simulink model "ADMIRE"  (R2021b)
settings: Solver=ode4  StartTime=0.0  StopTime=100  FixedStep=1e-2  RelTol=1e-3
undefined symbols (not defined in the file or in its folder): admireDB, Earth, WGS84
libraries: simulink_extras x112, simulink x27, aerolibutil x4, dspsigops x4, aerolibfltsims x3, sharedtransform x2, aerolibtransform2 x2, aerolibatmos2 x1, matrix_library x1, sharedutil x1, aerolibanimutils x1, vrlib x1
(part 13 of 15)

== system ADMIRE/Aircraft/Aerodynamics/RollMomentCoefficient/MachRegion3/Crmdr/Crmdr_ ==
  qacorr : Inport
  mach_nd : Inport  Port=2
  dR : Inport  Port=3
  CRMDRM_M : Lookup_n-D  NumberOfTableDimensions=1  BreakpointsForDimension1=admireDB.aerodata_asym_ext.CRMDRM.breakpoints.M  BreakpointsForDimension3=[5, 7]  Table=admireDB.aerodata_asym_ext.CRMDRM.newTable  ExtrapMethod=Clip  InternalRulePriority=Speed  RndMeth=Simplest  InputSameDT=on
  CRMEDR_QA_M : Lookup_n-D  BreakpointsForDimension1=admireDB.aerodata_asym_ext.CRMEDR.breakpoints.M  BreakpointsForDimension2=admireDB.aerodata_asym_ext.CRMEDR.breakpoints.QA  BreakpointsForDimension3=[5, 7]  Table=admireDB.aerodata_asym_ext.CRMEDR.newTable  ExtrapMethod=Clip  InternalRulePriority=Speed  RndMeth=Simplest  InputSameDT=on
      settings: InputPortMap=u0,u1
  Degrees to Radians : simulink_extras/Transformations/Degrees to Radians
  Product2 : Product  Inputs=3
  Crmdr : Outport
  wires:
  dR/1 -> Degrees to Radians/1
  CRMDRM_M/1 -> Product2/1
  Degrees to Radians/1 -> Product2/2
  qacorr/1 -> CRMEDR_QA_M/2
  mach_nd/1 -> CRMEDR_QA_M/1, CRMDRM_M/1
  CRMEDR_QA_M/1 -> Product2/3
  Product2/1 -> Crmdr/1

== system ADMIRE/Aircraft/Aerodynamics/RollMomentCoefficient/MachRegion3/Crmp/Crmp_ ==
  angleOfAttack_deg : Inport
  mach_nd : Inport  Port=2
  pc : Inport  Port=3
  qacorr : Inport  Port=4
  CRMEP_QA_M : Lookup_n-D  BreakpointsForDimension1=admireDB.aerodata_asym_ext.CRMEP.breakpoints.M  BreakpointsForDimension2=admireDB.aerodata_asym_ext.CRMEP.breakpoints.QA  BreakpointsForDimension3=[5, 7]  Table=admireDB.aerodata_asym_ext.CRMEP.newTable  ExtrapMethod=Clip  InternalRulePriority=Speed  RndMeth=Simplest  InputSameDT=on
      settings: InputPortMap=u0,u1
  CRMPAM_ALFA_M : Lookup_n-D  BreakpointsForDimension1=admireDB.aerodata_asym_ext.CRMPAM.breakpoints.M  BreakpointsForDimension2=admireDB.aerodata_asym_ext.CRMPAM.breakpoints.ALFA  BreakpointsForDimension3=[5, 7]  Table=admireDB.aerodata_asym_ext.CRMPAM.newTable  ExtrapMethod=Clip  InternalRulePriority=Speed  RndMeth=Simplest  InputSameDT=on
      settings: InputPortMap=u0,u1
  Product : Product  Inputs=3
  Crmp : Outport
  wires:
  qacorr/1 -> CRMEP_QA_M/2
  CRMPAM_ALFA_M/1 -> Product/1
  angleOfAttack_deg/1 -> CRMPAM_ALFA_M/2
  Product/1 -> Crmp/1
  pc/1 -> Product/2
  CRMEP_QA_M/1 -> Product/3
  mach_nd/1 -> CRMPAM_ALFA_M/1, CRMEP_QA_M/1

== system ADMIRE/Aircraft/Aerodynamics/RollMomentCoefficient/MachRegion3/Crmr/Crmr_ ==
  angleOfAttack_deg : Inport
  mach_nd : Inport  Port=2
  rc : Inport  Port=3
  CRMRAM_ALFA_M : Lookup_n-D  BreakpointsForDimension1=admireDB.aerodata_asym_ext.CRMRAM.breakpoints.M  BreakpointsForDimension2=admireDB.aerodata_asym_ext.CRMRAM.breakpoints.ALFA  BreakpointsForDimension3=[5, 7]  Table=admireDB.aerodata_asym_ext.CRMRAM.newTable  ExtrapMethod=Clip  InternalRulePriority=Speed  RndMeth=Simplest  InputSameDT=on
      settings: InputPortMap=u0,u1
  Product : Product  Inputs=**
  Crmr : Outport
  wires:
  CRMRAM_ALFA_M/1 -> Product/1
  mach_nd/1 -> CRMRAM_ALFA_M/1
  angleOfAttack_deg/1 -> CRMRAM_ALFA_M/2
  Product/1 -> Crmr/1
  rc/1 -> Product/2

== system ADMIRE/Aircraft/Aerodynamics/RollMomentCoefficient/MachRegion3/Crmrde/Crmrde_ ==
  mach_nd : Inport
  angleOfAttack_deg : Inport  Port=2
  rc : Inport  Port=3
  dEI : Inport  Port=4
  eieff : Inport  Port=5
  dEY : Inport  Port=6
  eoeff : Inport  Port=7
  CRMRDEM_M : Lookup_n-D  NumberOfTableDimensions=1  BreakpointsForDimension1=admireDB.aerodata_asym_ext.CRMRDEM.breakpoints.M  BreakpointsForDimension3=[5, 7]  Table=admireDB.aerodata_asym_ext.CRMRDEM.newTable  ExtrapMethod=Clip  InternalRulePriority=Speed  RndMeth=Simplest  InputSameDT=on
  CRMRKA_ALFA : Lookup_n-D  NumberOfTableDimensions=1  BreakpointsForDimension1=admireDB.aerodata_asym_ext.CRMRKA.breakpoints.ALFA  BreakpointsForDimension3=[5, 7]  Table=admireDB.aerodata_asym_ext.CRMRKA.newTable  ExtrapMethod=Clip  InternalRulePriority=Speed  RndMeth=Simplest  InputSameDT=on
  Constant : Constant  Value=1/30
  Constant1 : Constant  Value=1/30
  Product : Product  Inputs=****
  Product1 : Product  Inputs=3
  Product2 : Product  Inputs=3
  Sum : Sum  Inputs=|++
  Crmrde : Outport
  wires:
  Sum/1 -> Product/4
  Product2/1 -> Sum/2
  Product1/1 -> Sum/1
  dEY/1 -> Product2/1
  eoeff/1 -> Product2/3
  Constant1/1 -> Product2/2
  Constant/1 -> Product1/2
  eieff/1 -> Product1/3
  dEI/1 -> Product1/1
  CRMRKA_ALFA/1 -> Product/2
  CRMRDEM_M/1 -> Product/1
  mach_nd/1 -> CRMRDEM_M/1
  angleOfAttack_deg/1 -> CRMRKA_ALFA/1
  Product/1 -> Crmrde/1
  rc/1 -> Product/3

== system ADMIRE/Aircraft/Aerodynamics/RollMomentCoefficient/MachRegion4/Crmbde/Crmbde_ ==
  angleOfAttack_deg : Inport
  dN : Inport  Port=2
  dEI : Inport  Port=3
  angleOfSideslip_deg : Inport  Port=4
  dEY : Inport  Port=5
  eieff : Inport  Port=6
  eoeff : Inport  Port=7
  mach_nd : Inport  Port=8
  Abs : Abs
  CRMBKM_M : Lookup_n-D  NumberOfTableDimensions=1  BreakpointsForDimension1=admireDB.aerodata_asym_ext.CRMBKM.breakpoints.M  BreakpointsForDimension3=[5, 7]  Table=admireDB.aerodata_asym_ext.CRMBKM.newTable  ExtrapMethod=Clip  InternalRulePriority=Speed  RndMeth=Simplest  InputSameDT=on
  CRMDEB_ALFA_DN_DE_BETA : Lookup_n-D  NumberOfTableDimensions=4  BreakpointsForDimension1=admireDB.aerodata_asym_ext.CRMDEB.breakpoints.ALFA  BreakpointsForDimension2=admireDB.aerodata_asym_ext.CRMDEB.breakpoints.DN  BreakpointsForDimension3=admireDB.aerodata_asym_ext.CRMDEB.breakpoints.DE  BreakpointsForDimension4=admireDB.aerodata_asym_ext.CRMDEB.breakpoints.BETA  Table=admireDB.aerodata_asym_ext.CRMDEB.newTable  ExtrapMethod=Clip  InternalRulePriority=Speed  RndMeth=Simplest  InputSameDT=on
      settings: InputPortMap=u0,u1,u2,u3
  CRMDEB_ALFA_DN_DE_BETA1 : Lookup_n-D  NumberOfTableDimensions=4  BreakpointsForDimension1=admireDB.aerodata_asym_ext.CRMDEB.breakpoints.ALFA  BreakpointsForDimension2=admireDB.aerodata_asym_ext.CRMDEB.breakpoints.DN  BreakpointsForDimension3=admireDB.aerodata_asym_ext.CRMDEB.breakpoints.DE  BreakpointsForDimension4=admireDB.aerodata_asym_ext.CRMDEB.breakpoints.BETA  Table=admireDB.aerodata_asym_ext.CRMDEB.newTable  ExtrapMethod=Clip  InternalRulePriority=Speed  RndMeth=Simplest  InputSameDT=on
      settings: InputPortMap=u0,u1,u2,u3
  Product : Product  Inputs=**
  Product1 : Product  Inputs=**
  Product2 : Product  Inputs=3
  Sign : Signum
  Sum : Sum  Inputs=|++
  Crmbde : Outport
  wires:
  dEY/1 -> CRMDEB_ALFA_DN_DE_BETA1/3
  angleOfAttack_deg/1 -> CRMDEB_ALFA_DN_DE_BETA1/1, CRMDEB_ALFA_DN_DE_BETA/1
  dN/1 -> CRMDEB_ALFA_DN_DE_BETA/2, CRMDEB_ALFA_DN_DE_BETA1/2
  dEI/1 -> CRMDEB_ALFA_DN_DE_BETA/3
  Abs/1 -> CRMDEB_ALFA_DN_DE_BETA/4, CRMDEB_ALFA_DN_DE_BETA1/4
  CRMBKM_M/1 -> Product2/3
  mach_nd/1 -> CRMBKM_M/1
  Sign/1 -> Product2/1
  Product2/1 -> Crmbde/1
  Product1/1 -> Sum/2
  Product/1 -> Sum/1
  Sum/1 -> Product2/2
  eoeff/1 -> Product1/1
  eieff/1 -> Product/2
  CRMDEB_ALFA_DN_DE_BETA1/1 -> Product1/2
  CRMDEB_ALFA_DN_DE_BETA/1 -> Product/1
  angleOfSideslip_deg/1 -> Sign/1, Abs/1

== system ADMIRE/Aircraft/Aerodynamics/RollMomentCoefficient/MachRegion4/Crmbdle/Crmbdle_ ==
  angleOfAttack_deg : Inport
  dEI : Inport  Port=2
  mach_nd : Inport  Port=3
  dEY : Inport  Port=4
  eieff : Inport  Port=5
  eoeff : Inport  Port=6
  angleOfSideslip_deg : Inport  Port=7
  dLE : Inport  Port=8
  CRMBDLE_ALFA_DE_M : Lookup_n-D  NumberOfTableDimensions=3  BreakpointsForDimension1=admireDB.aerodata_asym_ext.CRMBDLE.breakpoints.ALFA  BreakpointsForDimension2=admireDB.aerodata_asym_ext.CRMBDLE.breakpoints.DE  BreakpointsForDimension3=admireDB.aerodata_asym_ext.CRMBDLE.breakpoints.M  Table=admireDB.aerodata_asym_ext.CRMBDLE.newTable  ExtrapMethod=Clip  InternalRulePriority=Speed  RndMeth=Simplest  InputSameDT=on
      settings: InputPortMap=u0,u1,u2
  CRMBDLE_ALFA_DE_M1 : Lookup_n-D  NumberOfTableDimensions=3  BreakpointsForDimension1=admireDB.aerodata_asym_ext.CRMBDLE.breakpoints.ALFA  BreakpointsForDimension2=admireDB.aerodata_asym_ext.CRMBDLE.breakpoints.DE  BreakpointsForDimension3=admireDB.aerodata_asym_ext.CRMBDLE.breakpoints.M  Table=admireDB.aerodata_asym_ext.CRMBDLE.newTable  ExtrapMethod=Clip  InternalRulePriority=Speed  RndMeth=Simplest  InputSameDT=on
      settings: InputPortMap=u0,u1,u2
  Constant : Constant  Value=1/27
  Degrees to Radians : simulink_extras/Transformations/Degrees to Radians
  Product : Product  Inputs=**
  Product1 : Product  Inputs=**
  Product2 : Product  Inputs=****
  Sum : Sum  Inputs=|++
  Crmbdle : Outport
  wires:
  dEY/1 -> CRMBDLE_ALFA_DE_M1/2
  dEI/1 -> CRMBDLE_ALFA_DE_M/2
  mach_nd/1 -> CRMBDLE_ALFA_DE_M/3, CRMBDLE_ALFA_DE_M1/3
  angleOfAttack_deg/1 -> CRMBDLE_ALFA_DE_M/1, CRMBDLE_ALFA_DE_M1/1
  Product2/1 -> Crmbdle/1
  Constant/1 -> Product2/4
  Sum/1 -> Product2/2
  Product1/1 -> Sum/2
  Product/1 -> Sum/1
  dLE/1 -> Product2/3
  Degrees to Radians/1 -> Product2/1
  angleOfSideslip_deg/1 -> Degrees to Radians/1
  CRMBDLE_ALFA_DE_M1/1 -> Product1/1
  eoeff/1 -> Product1/2
  CRMBDLE_ALFA_DE_M/1 -> Product/1
  eieff/1 -> Product/2

== system ADMIRE/Aircraft/Aerodynamics/RollMomentCoefficient/MachRegion4/Crmbdn/Crmbdn_ ==
  dN : Inport
  mach_nd : Inport  Port=2
  angleOfSideslip_deg : Inport  Port=3
  CRMBMDN_DN_M : Lookup_n-D  BreakpointsForDimension1=admireDB.aerodata_asym_ext.CRMBMDN.breakpoints.M  BreakpointsForDimension2=admireDB.aerodata_asym_ext.CRMBMDN.breakpoints.DN  BreakpointsForDimension3=[5, 7]  Table=admireDB.aerodata_asym_ext.CRMBMDN.newTable  ExtrapMethod=Clip  InternalRulePriority=Speed  RndMeth=Simplest  InputSameDT=on
      settings: InputPortMap=u0,u1
  Degrees to Radians : simulink_extras/Transformations/Degrees to Radians
  Product : Product  Inputs=**
  Crmbdn : Outport
  wires:
  Product/1 -> Crmbdn/1
  CRMBMDN_DN_M/1 -> Product/1
  angleOfSideslip_deg/1 -> Degrees to Radians/1
  mach_nd/1 -> CRMBMDN_DN_M/1
  Degrees to Radians/1 -> Product/2
  dN/1 -> CRMBMDN_DN_M/2

== system ADMIRE/Aircraft/Aerodynamics/RollMomentCoefficient/MachRegion4/Crmbeta/Crmbeta_ ==
  mach_nd : Inport
  angleOfAttack_deg : Inport  Port=2
  angleOfSideslip_deg : Inport  Port=3
  qacorr : Inport  Port=4
  CRMBMA_M_ALFA : Lookup_n-D  BreakpointsForDimension1=admireDB.aerodata_asym_ext.CRMBMA.breakpoints.ALFA  BreakpointsForDimension2=admireDB.aerodata_asym_ext.CRMBMA.breakpoints.M  BreakpointsForDimension3=[5, 7]  Table=admireDB.aerodata_asym_ext.CRMBMA.newTable  ExtrapMethod=Clip  InternalRulePriority=Speed  RndMeth=Simplest  InputSameDT=on
      settings: InputPortMap=u0,u1
  CRMEB_QA_M : Lookup_n-D  BreakpointsForDimension1=admireDB.aerodata_asym_ext.CRMEB.breakpoints.M  BreakpointsForDimension2=admireDB.aerodata_asym_ext.CRMEB.breakpoints.QA  BreakpointsForDimension3=[5, 7]  Table=admireDB.aerodata_asym_ext.CRMEB.newTable  ExtrapMethod=Clip  InternalRulePriority=Speed  RndMeth=Simplest  InputSameDT=on
      settings: InputPortMap=u0,u1
  Degrees to Radians : simulink_extras/Transformations/Degrees to Radians
  Product1 : Product
  Sum : Sum  Inputs=|++
  Crmbeta : Outport
  wires:
  CRMBMA_M_ALFA/1 -> Sum/1
  mach_nd/1 -> CRMBMA_M_ALFA/2, CRMEB_QA_M/1
  angleOfAttack_deg/1 -> CRMBMA_M_ALFA/1
  qacorr/1 -> CRMEB_QA_M/2
  angleOfSideslip_deg/1 -> Degrees to Radians/1
  CRMEB_QA_M/1 -> Product1/2
  Degrees to Radians/1 -> Product1/1
  Product1/1 -> Sum/2
  Sum/1 -> Crmbeta/1

== system ADMIRE/Aircraft/Aerodynamics/RollMomentCoefficient/MachRegion4/Crmbetad/Crmbetad_ ==
  angleOfAttack_deg : Inport
  mach_nd : Inport  Port=2
  betad : Inport  Port=3
  CRMBDH_ALFA_M : Lookup_n-D  BreakpointsForDimension1=admireDB.aerodata_asym_ext.CRMBDH.breakpoints.M  BreakpointsForDimension2=admireDB.aerodata_asym_ext.CRMBDH.breakpoints.ALFA  BreakpointsForDimension3=[5, 7]  Table=admireDB.aerodata_asym_ext.CRMBDH.newTable  ExtrapMethod=Clip  InternalRulePriority=Speed  RndMeth=Simplest  InputSameDT=on
      settings: InputPortMap=u0,u1
  Product : Product  Inputs=**
  Crmbetad : Outport
  wires:
  CRMBDH_ALFA_M/1 -> Product/1
  angleOfAttack_deg/1 -> CRMBDH_ALFA_M/2
  mach_nd/1 -> CRMBDH_ALFA_M/1
  Product/1 -> Crmbetad/1
  betad/1 -> Product/2

== system ADMIRE/Aircraft/Aerodynamics/RollMomentCoefficient/MachRegion4/Crmblg/Crmblg_ ==
  dLG : Inport
  angleOfAttack_deg : Inport  Port=2
  angleOfSideslip_deg : Inport  Port=3
  CRMBLST_NG_DOOR_ALFA : Lookup_n-D  BreakpointsForDimension1=admireDB.aerodata_asym_ext.CRMBLST.breakpoints.ALFA  BreakpointsForDimension2=admireDB.aerodata_asym_ext.CRMBLST.breakpoints.NG_DOOR  BreakpointsForDimension3=[5, 7]  Table=admireDB.aerodata_asym_ext.CRMBLST.newTable  ExtrapMethod=Clip  InternalRulePriority=Speed  RndMeth=Simplest  InputSameDT=on
      settings: InputPortMap=u0,u1
  Degrees to Radians : simulink_extras/Transformations/Degrees to Radians
  Product : Product  Inputs=3
  Crmblg : Outport
  wires:
  Degrees to Radians/1 -> Product/3
  CRMBLST_NG_DOOR_ALFA/1 -> Product/2
  dLG/1 -> CRMBLST_NG_DOOR_ALFA/2, Product/1
  angleOfAttack_deg/1 -> CRMBLST_NG_DOOR_ALFA/1
  Product/1 -> Crmblg/1
  angleOfSideslip_deg/1 -> Degrees to Radians/1

== system ADMIRE/Aircraft/Aerodynamics/RollMomentCoefficient/MachRegion4/Crmdai/Crmdai_ ==
  angleOfAttack_deg : Inport
  dEI : Inport  Port=2
  mach_nd : Inport  Port=3
  dAI : Inport  Port=4
  eieff : Inport  Port=5
  qacorr : Inport  Port=6
  CRMDA_ALFA_DE_M : Lookup_n-D  NumberOfTableDimensions=3  BreakpointsForDimension1=admireDB.aerodata_asym_ext.CRMDA.breakpoints.ALFA  BreakpointsForDimension2=admireDB.aerodata_asym_ext.CRMDA.breakpoints.DE  BreakpointsForDimension3=admireDB.aerodata_asym_ext.CRMDA.breakpoints.M  Table=admireDB.aerodata_asym_ext.CRMDA.newTable  ExtrapMethod=Clip  InternalRulePriority=Speed  RndMeth=Simplest  InputSameDT=on
      settings: InputPortMap=u0,u1,u2
  CRMEDAI_QA_M : Lookup_n-D  BreakpointsForDimension1=admireDB.aerodata_asym_ext.CRMEDAI.breakpoints.M  BreakpointsForDimension2=admireDB.aerodata_asym_ext.CRMEDAI.breakpoints.QA  BreakpointsForDimension3=[5, 7]  Table=admireDB.aerodata_asym_ext.CRMEDAI.newTable  ExtrapMethod=Clip  InternalRulePriority=Speed  RndMeth=Simplest  InputSameDT=on
      settings: InputPortMap=u0,u1
  Degrees to Radians : simulink_extras/Transformations/Degrees to Radians
  Product1 : Product
  Product3 : Product  Inputs=***
  Crmdai : Outport
  wires:
  qacorr/1 -> CRMEDAI_QA_M/2
  angleOfAttack_deg/1 -> CRMDA_ALFA_DE_M/1
  dEI/1 -> CRMDA_ALFA_DE_M/2
  dAI/1 -> Degrees to Radians/1
  CRMDA_ALFA_DE_M/1 -> Product1/2
  Degrees to Radians/1 -> Product1/1
  Product1/1 -> Product3/1
  Product3/1 -> Crmdai/1
  mach_nd/1 -> CRMDA_ALFA_DE_M/3, CRMEDAI_QA_M/1
  CRMEDAI_QA_M/1 -> Product3/3
  eieff/1 -> Product3/2

== system ADMIRE/Aircraft/Aerodynamics/RollMomentCoefficient/MachRegion4/Crmday/Crmday_ ==
  angleOfAttack_deg : Inport
  dEY : Inport  Port=2
  mach_nd : Inport  Port=3
  dAY : Inport  Port=4
  eoeff : Inport  Port=5
  qacorr : Inport  Port=6
  CRMDA_ALFA_DE_M : Lookup_n-D  NumberOfTableDimensions=3  BreakpointsForDimension1=admireDB.aerodata_asym_ext.CRMDA.breakpoints.ALFA  BreakpointsForDimension2=admireDB.aerodata_asym_ext.CRMDA.breakpoints.DE  BreakpointsForDimension3=admireDB.aerodata_asym_ext.CRMDA.breakpoints.M  Table=admireDB.aerodata_asym_ext.CRMDA.newTable  ExtrapMethod=Clip  InternalRulePriority=Speed  RndMeth=Simplest  InputSameDT=on
      settings: InputPortMap=u0,u1,u2
  CRMEDAY_QA_M : Lookup_n-D  BreakpointsForDimension1=admireDB.aerodata_asym_ext.CRMEDAY.breakpoints.M  BreakpointsForDimension2=admireDB.aerodata_asym_ext.CRMEDAY.breakpoints.QA  BreakpointsForDimension3=[5, 7]  Table=admireDB.aerodata_asym_ext.CRMEDAY.newTable  ExtrapMethod=Clip  InternalRulePriority=Speed  RndMeth=Simplest  InputSameDT=on
      settings: InputPortMap=u0,u1
  Degrees to Radians : simulink_extras/Transformations/Degrees to Radians
  Product1 : Product
  Product3 : Product  Inputs=***
  Crmday : Outport
  wires:
  angleOfAttack_deg/1 -> CRMDA_ALFA_DE_M/1
  dEY/1 -> CRMDA_ALFA_DE_M/2
  dAY/1 -> Degrees to Radians/1
  CRMDA_ALFA_DE_M/1 -> Product1/2
  Degrees to Radians/1 -> Product1/1
  Product1/1 -> Product3/1
  Product3/1 -> Crmday/1
  qacorr/1 -> CRMEDAY_QA_M/2
  CRMEDAY_QA_M/1 -> Product3/3
  mach_nd/1 -> CRMDA_ALFA_DE_M/3, CRMEDAY_QA_M/1
  eoeff/1 -> Product3/2

== system ADMIRE/Aircraft/Aerodynamics/RollMomentCoefficient/MachRegion4/Crmdna/Crmdna_ ==
  angleOfAttack_deg : Inport
  dNA : Inport  Port=2
  CRMDNAAM_ALFA_M : Lookup_n-D  BreakpointsForDimension1=admireDB.aerodata_asym_ext.CRMDNAAM.breakpoints.M  BreakpointsForDimension2=admireDB.aerodata_asym_ext.CRMDNAAM.breakpoints.ALFA  BreakpointsForDimension3=[5, 7]  Table=admireDB.aerodata_asym_ext.CRMDNAAM.newTable  ExtrapMethod=Clip  InternalRulePriority=Speed  RndMeth=Simplest  InputSameDT=on
      settings: InputPortMap=u0,u1
  Degrees to Radians : simulink_extras/Transformations/Degrees to Radians
  Product : Product  Inputs=**
  mach_nd_cnst : Constant  Value=0.5
  Crmdna : Outport
  wires:
  Degrees to Radians/1 -> Product/2
  dNA/1 -> Degrees to Radians/1
  mach_nd_cnst/1 -> CRMDNAAM_ALFA_M/1
  Product/1 -> Crmdna/1
  angleOfAttack_deg/1 -> CRMDNAAM_ALFA_M/2
  CRMDNAAM_ALFA_M/1 -> Product/1

== system ADMIRE/Aircraft/Aerodynamics/RollMomentCoefficient/MachRegion4/Crmdr/Crmdr_ ==
  qacorr : Inport
  mach_nd : Inport  Port=2
  dR : Inport  Port=3
  CRMDRM_M : Lookup_n-D  NumberOfTableDimensions=1  BreakpointsForDimension1=admireDB.aerodata_asym_ext.CRMDRM.breakpoints.M  BreakpointsForDimension3=[5, 7]  Table=admireDB.aerodata_asym_ext.CRMDRM.newTable  ExtrapMethod=Clip  InternalRulePriority=Speed  RndMeth=Simplest  InputSameDT=on
  CRMEDR_QA_M : Lookup_n-D  BreakpointsForDimension1=admireDB.aerodata_asym_ext.CRMEDR.breakpoints.M  BreakpointsForDimension2=admireDB.aerodata_asym_ext.CRMEDR.breakpoints.QA  BreakpointsForDimension3=[5, 7]  Table=admireDB.aerodata_asym_ext.CRMEDR.newTable  ExtrapMethod=Clip  InternalRulePriority=Speed  RndMeth=Simplest  InputSameDT=on
      settings: InputPortMap=u0,u1
  Degrees to Radians : simulink_extras/Transformations/Degrees to Radians
  Product2 : Product  Inputs=3
  Crmdr : Outport
  wires:
  dR/1 -> Degrees to Radians/1
  CRMDRM_M/1 -> Product2/1
  Degrees to Radians/1 -> Product2/2
  qacorr/1 -> CRMEDR_QA_M/2
  mach_nd/1 -> CRMEDR_QA_M/1, CRMDRM_M/1
  CRMEDR_QA_M/1 -> Product2/3
  Product2/1 -> Crmdr/1

== system ADMIRE/Aircraft/Aerodynamics/RollMomentCoefficient/MachRegion4/Crmp/Crmp_ ==
  angleOfAttack_deg : Inport
  mach_nd : Inport  Port=2
  pc : Inport  Port=3
  qacorr : Inport  Port=4
  CRMEP_QA_M : Lookup_n-D  BreakpointsForDimension1=admireDB.aerodata_asym_ext.CRMEP.breakpoints.M  BreakpointsForDimension2=admireDB.aerodata_asym_ext.CRMEP.breakpoints.QA  BreakpointsForDimension3=[5, 7]  Table=admireDB.aerodata_asym_ext.CRMEP.newTable  ExtrapMethod=Clip  InternalRulePriority=Speed  RndMeth=Simplest  InputSameDT=on
      settings: InputPortMap=u0,u1
  CRMPAM_ALFA_M : Lookup_n-D  BreakpointsForDimension1=admireDB.aerodata_asym_ext.CRMPAM.breakpoints.M  BreakpointsForDimension2=admireDB.aerodata_asym_ext.CRMPAM.breakpoints.ALFA  BreakpointsForDimension3=[5, 7]  Table=admireDB.aerodata_asym_ext.CRMPAM.newTable  ExtrapMethod=Clip  InternalRulePriority=Speed  RndMeth=Simplest  InputSameDT=on
      settings: InputPortMap=u0,u1
  Product : Product  Inputs=3
  Crmp : Outport
  wires:
  CRMPAM_ALFA_M/1 -> Product/1
  angleOfAttack_deg/1 -> CRMPAM_ALFA_M/2
  Product/1 -> Crmp/1
  pc/1 -> Product/2
  CRMEP_QA_M/1 -> Product/3
  qacorr/1 -> CRMEP_QA_M/2
  mach_nd/1 -> CRMPAM_ALFA_M/1, CRMEP_QA_M/1

== system ADMIRE/Aircraft/Aerodynamics/RollMomentCoefficient/MachRegion4/Crmr/Crmr_ ==
  angleOfAttack_deg : Inport
  mach_nd : Inport  Port=2
  rc : Inport  Port=3
  CRMRAM_ALFA_M : Lookup_n-D  BreakpointsForDimension1=admireDB.aerodata_asym_ext.CRMRAM.breakpoints.M  BreakpointsForDimension2=admireDB.aerodata_asym_ext.CRMRAM.breakpoints.ALFA  BreakpointsForDimension3=[5, 7]  Table=admireDB.aerodata_asym_ext.CRMRAM.newTable  ExtrapMethod=Clip  InternalRulePriority=Speed  RndMeth=Simplest  InputSameDT=on
      settings: InputPortMap=u0,u1
  Product : Product  Inputs=**
  Crmr : Outport
  wires:
  CRMRAM_ALFA_M/1 -> Product/1
  angleOfAttack_deg/1 -> CRMRAM_ALFA_M/2
  mach_nd/1 -> CRMRAM_ALFA_M/1
  Product/1 -> Crmr/1
  rc/1 -> Product/2

== system ADMIRE/Aircraft/Aerodynamics/RollMomentCoefficient/MachRegion4/Crmrde/Crmrde_ ==
  mach_nd : Inport
  angleOfAttack_deg : Inport  Port=2
  rc : Inport  Port=3
  dEI : Inport  Port=4
  eieff : Inport  Port=5
  dEY : Inport  Port=6
  eoeff : Inport  Port=7
  CRMRDEM_M : Lookup_n-D  NumberOfTableDimensions=1  BreakpointsForDimension1=admireDB.aerodata_asym_ext.CRMRDEM.breakpoints.M  BreakpointsForDimension3=[5, 7]  Table=admireDB.aerodata_asym_ext.CRMRDEM.newTable  ExtrapMethod=Clip  InternalRulePriority=Speed  RndMeth=Simplest  InputSameDT=on
  CRMRKA_ALFA : Lookup_n-D  NumberOfTableDimensions=1  BreakpointsForDimension1=admireDB.aerodata_asym_ext.CRMRKA.breakpoints.ALFA  BreakpointsForDimension3=[5, 7]  Table=admireDB.aerodata_asym_ext.CRMRKA.newTable  ExtrapMethod=Clip  InternalRulePriority=Speed  RndMeth=Simplest  InputSameDT=on
  Constant : Constant  Value=1/30
  Constant1 : Constant  Value=1/30
  Product : Product  Inputs=****
  Product1 : Product  Inputs=3
  Product2 : Product  Inputs=3
  Sum : Sum  Inputs=|++
  Crmrde : Outport
  wires:
  Sum/1 -> Product/4
  Product2/1 -> Sum/2
  Product1/1 -> Sum/1
  dEY/1 -> Product2/1
  eoeff/1 -> Product2/3
  Constant1/1 -> Product2/2
  Constant/1 -> Product1/2
  eieff/1 -> Product1/3
  dEI/1 -> Product1/1
  CRMRKA_ALFA/1 -> Product/2
  CRMRDEM_M/1 -> Product/1
  mach_nd/1 -> CRMRDEM_M/1
  angleOfAttack_deg/1 -> CRMRKA_ALFA/1
  Product/1 -> Crmrde/1
  rc/1 -> Product/3

== system ADMIRE/Aircraft/Aerodynamics/YawMomentCoefficient/MachRegion1/Cymbasic/Cymbasic_ ==
  angleOfAttack_deg : Inport
  Abs : Abs
  CYMZERO_ALFA : Lookup_n-D  NumberOfTableDimensions=1  BreakpointsForDimension1=admireDB.aerodata_asym_ext.CYMZERO.breakpoints.ALFA  BreakpointsForDimension3=[5, 7]  Table=admireDB.aerodata_asym_ext.CYMZERO.newTable  ExtrapMethod=Clip  InternalRulePriority=Speed  RndMeth=Simplest  InputSameDT=on
  Cymbasic : Outport
  wires:
  CYMZERO_ALFA/1 -> Cymbasic/1
  angleOfAttack_deg/1 -> Abs/1
  Abs/1 -> CYMZERO_ALFA/1

== system ADMIRE/Aircraft/Aerodynamics/YawMomentCoefficient/MachRegion1/Cymbcai/Cymbcai_ ==
  CAI : Inport
  angleOfAttack_deg : Inport  Port=2
  angleOfSideslip_deg : Inport  Port=3
  CYMBCAI_CAI_ALFA : Lookup_n-D  BreakpointsForDimension1=admireDB.aerodata_asym_ext.CYMBCAI.breakpoints.ALFA  BreakpointsForDimension2=admireDB.aerodata_asym_ext.CYMBCAI.breakpoints.CAI  BreakpointsForDimension3=[5, 7]  Table=admireDB.aerodata_asym_ext.CYMBCAI.newTable  ExtrapMethod=Clip  InternalRulePriority=Speed  RndMeth=Simplest  InputSameDT=on
      settings: InputPortMap=u0,u1
  Degrees to Radians : simulink_extras/Transformations/Degrees to Radians
  Product : Product  Inputs=**
  Cymbcai : Outport
  wires:
  Product/1 -> Cymbcai/1
  CYMBCAI_CAI_ALFA/1 -> Product/1
  angleOfAttack_deg/1 -> CYMBCAI_CAI_ALFA/1
  Degrees to Radians/1 -> Product/2
  angleOfSideslip_deg/1 -> Degrees to Radians/1
  CAI/1 -> CYMBCAI_CAI_ALFA/2

== system ADMIRE/Aircraft/Aerodynamics/YawMomentCoefficient/MachRegion1/Cymbde/Cymbde_ ==
  angleOfAttack_deg : Inport
  dEI : Inport  Port=2
  angleOfSideslip_deg : Inport  Port=3
  dEY : Inport  Port=4
  eieff : Inport  Port=5
  eoeff : Inport  Port=6
  Abs : Abs
  CYMDEB_ALFA_DE_BETA : Lookup_n-D  NumberOfTableDimensions=3  BreakpointsForDimension1=admireDB.aerodata_asym_ext.CYMDEB.breakpoints.ALFA  BreakpointsForDimension2=admireDB.aerodata_asym_ext.CYMDEB.breakpoints.DE  BreakpointsForDimension3=admireDB.aerodata_asym_ext.CYMDEB.breakpoints.BETA  Table=admireDB.aerodata_asym_ext.CYMDEB.newTable  ExtrapMethod=Clip  InternalRulePriority=Speed  RndMeth=Simplest  InputSameDT=on
      settings: InputPortMap=u0,u1,u2
  CYMDEB_ALFA_DE_BETA1 : Lookup_n-D  NumberOfTableDimensions=3  BreakpointsForDimension1=admireDB.aerodata_asym_ext.CYMDEB.breakpoints.ALFA  BreakpointsForDimension2=admireDB.aerodata_asym_ext.CYMDEB.breakpoints.DE  BreakpointsForDimension3=admireDB.aerodata_asym_ext.CYMDEB.breakpoints.BETA  Table=admireDB.aerodata_asym_ext.CYMDEB.newTable  ExtrapMethod=Clip  InternalRulePriority=Speed  RndMeth=Simplest  InputSameDT=on
      settings: InputPortMap=u0,u1,u2
  Product : Product  Inputs=**
  Product1 : Product  Inputs=**
  Product2 : Product  Inputs=**
  Sign : Signum
  Sum : Sum  Inputs=|++
  Cymbde : Outport
  wires:
  Abs/1 -> CYMDEB_ALFA_DE_BETA/3, CYMDEB_ALFA_DE_BETA1/3
  Product2/1 -> Cymbde/1
  Sign/1 -> Product2/1
  Product1/1 -> Sum/2
  eoeff/1 -> Product1/2
  CYMDEB_ALFA_DE_BETA1/1 -> Product1/1
  dEY/1 -> CYMDEB_ALFA_DE_BETA1/2
  Sum/1 -> Product2/2
  Product/1 -> Sum/1
  angleOfAttack_deg/1 -> CYMDEB_ALFA_DE_BETA/1, CYMDEB_ALFA_DE_BETA1/1
  eieff/1 -> Product/2
  CYMDEB_ALFA_DE_BETA/1 -> Product/1
  angleOfSideslip_deg/1 -> Abs/1, Sign/1
  dEI/1 -> CYMDEB_ALFA_DE_BETA/2

== system ADMIRE/Aircraft/Aerodynamics/YawMomentCoefficient/MachRegion1/Cymbdle/Cymbdle_ ==
  angleOfAttack_deg : Inport
  dEI : Inport  Port=2
  angleOfSideslip_deg : Inport  Port=3
  dLE : Inport  Port=4
  dEY : Inport  Port=5
  eieff : Inport  Port=6
  eoeff : Inport  Port=7
  Abs : Abs
  CYMDLEB_ALFA_DE_BETA_DLE : Lookup_n-D  NumberOfTableDimensions=4  BreakpointsForDimension1=admireDB.aerodata_asym_ext.CYMDLEB.breakpoints.ALFA  BreakpointsForDimension2=admireDB.aerodata_asym_ext.CYMDLEB.breakpoints.DE  BreakpointsForDimension3=admireDB.aerodata_asym_ext.CYMDLEB.breakpoints.BETA  BreakpointsForDimension4=admireDB.aerodata_asym_ext.CYMDLEB.breakpoints.DLE  Table=admireDB.aerodata_asym_ext.CYMDLEB.newTable  ExtrapMethod=Clip  InternalRulePriority=Speed  RndMeth=Simplest  InputSameDT=on
      settings: InputPortMap=u0,u1,u2,u3
  CYMDLEB_ALFA_DE_BETA_DLE1 : Lookup_n-D  NumberOfTableDimensions=4  BreakpointsForDimension1=admireDB.aerodata_asym_ext.CYMDLEB.breakpoints.ALFA  BreakpointsForDimension2=admireDB.aerodata_asym_ext.CYMDLEB.breakpoints.DE  BreakpointsForDimension3=admireDB.aerodata_asym_ext.CYMDLEB.breakpoints.BETA  BreakpointsForDimension4=admireDB.aerodata_asym_ext.CYMDLEB.breakpoints.DLE  Table=admireDB.aerodata_asym_ext.CYMDLEB.newTable  ExtrapMethod=Clip  InternalRulePriority=Speed  RndMeth=Simplest  InputSameDT=on
      settings: InputPortMap=u0,u1,u2,u3
  Product : Product  Inputs=**
  Product1 : Product  Inputs=**
  Product2 : Product
  Sign : Signum
  Sum : Sum  Inputs=|++
  Cymbdle : Outport
  wires:
  Product2/1 -> Cymbdle/1
  Sum/1 -> Product2/1
  Sign/1 -> Product2/2
  Product1/1 -> Sum/2
  Product/1 -> Sum/1
  eoeff/1 -> Product1/2
  CYMDLEB_ALFA_DE_BETA_DLE1/1 -> Product1/1
  dEY/1 -> CYMDLEB_ALFA_DE_BETA_DLE1/2
  Abs/1 -> CYMDLEB_ALFA_DE_BETA_DLE/3, CYMDLEB_ALFA_DE_BETA_DLE1/3
  angleOfAttack_deg/1 -> CYMDLEB_ALFA_DE_BETA_DLE/1, CYMDLEB_ALFA_DE_BETA_DLE1/1
  dLE/1 -> CYMDLEB_ALFA_DE_BETA_DLE/4, CYMDLEB_ALFA_DE_BETA_DLE1/4
  eieff/1 -> Product/2
  CYMDLEB_ALFA_DE_BETA_DLE/1 -> Product/1
  angleOfSideslip_deg/1 -> Abs/1, Sign/1
  dEI/1 -> CYMDLEB_ALFA_DE_BETA_DLE/2

== system ADMIRE/Aircraft/Aerodynamics/YawMomentCoefficient/MachRegion1/Cymbdn/Cymbdn_ ==
  angleOfAttack_deg : Inport
  dN : Inport  Port=2
  angleOfSideslip_deg : Inport  Port=3
  Abs : Abs
  CYMDNB_ALFA_DN_BETA : Lookup_n-D  NumberOfTableDimensions=3  BreakpointsForDimension1=admireDB.aerodata_asym_ext.CYMDNB.breakpoints.ALFA  BreakpointsForDimension2=admireDB.aerodata_asym_ext.CYMDNB.breakpoints.DN  BreakpointsForDimension3=admireDB.aerodata_asym_ext.CYMDNB.breakpoints.BETA  Table=admireDB.aerodata_asym_ext.CYMDNB.newTable  ExtrapMethod=Clip  InternalRulePriority=Speed  RndMeth=Simplest  InputSameDT=on
      settings: InputPortMap=u0,u1,u2
  Product : Product  Inputs=**
  Sign : Signum
  Cymbdn : Outport
  wires:
  Abs/1 -> CYMDNB_ALFA_DN_BETA/3
  Product/1 -> Cymbdn/1
  angleOfSideslip_deg/1 -> Sign/1, Abs/1
  CYMDNB_ALFA_DN_BETA/1 -> Product/1
  angleOfAttack_deg/1 -> CYMDNB_ALFA_DN_BETA/1
  Sign/1 -> Product/2
  dN/1 -> CYMDNB_ALFA_DN_BETA/2

== system ADMIRE/Aircraft/Aerodynamics/YawMomentCoefficient/MachRegion1/Cymbeta/Cymbeta_ ==
  angleOfSideslip_deg : Inport
  angleOfAttack_deg : Inport  Port=2
  qacorr : Inport  Port=3
  mach_nd : Inport  Port=4
  Abs : Abs
  CYMBAL_BETA_ALFA : Lookup_n-D  BreakpointsForDimension1=admireDB.aerodata_asym_ext.CYMBAL.breakpoints.ALFA  BreakpointsForDimension2=admireDB.aerodata_asym_ext.CYMBAL.breakpoints.BETA  BreakpointsForDimension3=[5, 7]  Table=admireDB.aerodata_asym_ext.CYMBAL.newTable  ExtrapMethod=Clip  InternalRulePriority=Speed  RndMeth=Simplest  InputSameDT=on
      settings: InputPortMap=u0,u1
  CYMEB_QA_M : Lookup_n-D  BreakpointsForDimension1=admireDB.aerodata_asym_ext.CYMEB.breakpoints.M  BreakpointsForDimension2=admireDB.aerodata_asym_ext.CYMEB.breakpoints.QA  BreakpointsForDimension3=[5, 7]  Table=admireDB.aerodata_asym_ext.CYMEB.newTable  ExtrapMethod=Clip  InternalRulePriority=Speed  RndMeth=Simplest  InputSameDT=on
      settings: InputPortMap=u0,u1
  Degrees to Radians : simulink_extras/Transformations/Degrees to Radians
  Product : Product
  Product1 : Product
  Sign : Signum
  Sum : Sum  Inputs=|++
  Cymbeta : Outport
  wires:
  Sum/1 -> Cymbeta/1
  qacorr/1 -> CYMEB_QA_M/2
  angleOfAttack_deg/1 -> CYMBAL_BETA_ALFA/1
  mach_nd/1 -> CYMEB_QA_M/1
  angleOfSideslip_deg/1 -> Abs/1, Sign/1, Degrees to Radians/1
  CYMBAL_BETA_ALFA/1 -> Product/2
  Sign/1 -> Product/1
  Abs/1 -> CYMBAL_BETA_ALFA/2
  CYMEB_QA_M/1 -> Product1/2
  Degrees to Radians/1 -> Product1/1
  Product1/1 -> Sum/2
  Product/1 -> Sum/1

== system ADMIRE/Aircraft/Aerodynamics/YawMomentCoefficient/MachRegion1/Cymbetad/Cymbetad_ ==
  angleOfAttack_deg : Inport
  betad : Inport  Port=2
  CYMBDL_ALFA : Lookup_n-D  NumberOfTableDimensions=1  BreakpointsForDimension1=admireDB.aerodata_asym_ext.CYMBDL.breakpoints.ALFA  BreakpointsForDimension3=[5, 7]  Table=admireDB.aerodata_asym_ext.CYMBDL.newTable  ExtrapMethod=Clip  InternalRulePriority=Speed  RndMeth=Simplest  InputSameDT=on
  Product : Product  Inputs=**
  Cymbetad : Outport
  wires:
  betad/1 -> Product/2
  CYMBDL_ALFA/1 -> Product/1
  Product/1 -> Cymbetad/1
  angleOfAttack_deg/1 -> CYMBDL_ALFA/1

== system ADMIRE/Aircraft/Aerodynamics/YawMomentCoefficient/MachRegion1/Cymblg/Cymblg_ ==
  angleOfSideslip_deg : Inport
  dLG : Inport  Port=2
  angleOfAttack_deg : Inport  Port=3
  CYMBLST_NG_DOOR_ALFA : Lookup_n-D  BreakpointsForDimension1=admireDB.aerodata_asym_ext.CYMBLST.breakpoints.ALFA  BreakpointsForDimension2=admireDB.aerodata_asym_ext.CYMBLST.breakpoints.NG_DOOR  BreakpointsForDimension3=[5, 7]  Table=admireDB.aerodata_asym_ext.CYMBLST.newTable  ExtrapMethod=Clip  InternalRulePriority=Speed  RndMeth=Simplest  InputSameDT=on
      settings: InputPortMap=u0,u1
  Degrees to Radians : simulink_extras/Transformations/Degrees to Radians
  Product : Product  Inputs=***
  Cymblg : Outport
  wires:
  angleOfSideslip_deg/1 -> Degrees to Radians/1
  CYMBLST_NG_DOOR_ALFA/1 -> Product/3
  Degrees to Radians/1 -> Product/1
  angleOfAttack_deg/1 -> CYMBLST_NG_DOOR_ALFA/1
  dLG/1 -> Product/2, CYMBLST_NG_DOOR_ALFA/2
  Product/1 -> Cymblg/1

== system ADMIRE/Aircraft/Aerodynamics/YawMomentCoefficient/MachRegion1/Cymdai/Cymdai_ ==
  dAI : Inport
  angleOfAttack_deg : Inport  Port=2
  dEI : Inport  Port=3
  eieff : Inport  Port=4
  qacorr : Inport  Port=5
  mach_nd : Inport  Port=6
  Abs : Abs
  CYMDAAL_DA_ALFA : Lookup_n-D  BreakpointsForDimension1=admireDB.aerodata_asym_ext.CYMDAAL.breakpoints.ALFA  BreakpointsForDimension2=admireDB.aerodata_asym_ext.CYMDAAL.breakpoints.DA  BreakpointsForDimension3=[5, 7]  Table=admireDB.aerodata_asym_ext.CYMDAAL.newTable  ExtrapMethod=Clip  InternalRulePriority=Speed  RndMeth=Simplest  InputSameDT=on
      settings: InputPortMap=u0,u1
  CYMDAL_DE_ALFA : Lookup_n-D  BreakpointsForDimension1=admireDB.aerodata_asym_ext.CYMDAL.breakpoints.ALFA  BreakpointsForDimension2=admireDB.aerodata_asym_ext.CYMDAL.breakpoints.DE  BreakpointsForDimension3=[5, 7]  Table=admireDB.aerodata_asym_ext.CYMDAL.newTable  ExtrapMethod=Clip  InternalRulePriority=Speed  RndMeth=Simplest  InputSameDT=on
      settings: InputPortMap=u0,u1
  CYMDAL_DE_ALFA1 : Lookup_n-D  BreakpointsForDimension1=admireDB.aerodata_asym_ext.CYMDAL.breakpoints.ALFA  BreakpointsForDimension2=admireDB.aerodata_asym_ext.CYMDAL.breakpoints.DE  BreakpointsForDimension3=[5, 7]  Table=admireDB.aerodata_asym_ext.CYMDAL.newTable  ExtrapMethod=Clip  InternalRulePriority=Speed  RndMeth=Simplest  InputSameDT=on
      settings: InputPortMap=u0,u1
  CYMEDAI_QA_M : Lookup_n-D  BreakpointsForDimension1=admireDB.aerodata_asym_ext.CYMEDAI.breakpoints.M  BreakpointsForDimension2=admireDB.aerodata_asym_ext.CYMEDAI.breakpoints.QA  BreakpointsForDimension3=[5, 7]  Table=admireDB.aerodata_asym_ext.CYMEDAI.newTable  ExtrapMethod=Clip  InternalRulePriority=Speed  RndMeth=Simplest  InputSameDT=on
      settings: InputPortMap=u0,u1
  Degrees to Radians : simulink_extras/Transformations/Degrees to Radians
  Product : Product
  Product1 : Product
  Product2 : Product  Inputs=3
  Sign : Signum
  Sum : Sum  Inputs=|+-
  Sum1 : Sum  Inputs=|++
  dE_cnst : Constant  Value=0.0
  Cymdai : Outport
  wires:
  dEI/1 -> CYMDAL_DE_ALFA/2
  dE_cnst/1 -> CYMDAL_DE_ALFA1/2
  Product2/1 -> Cymdai/1
  Abs/1 -> CYMDAAL_DA_ALFA/2
  dAI/1 -> Abs/1, Sign/1, Degrees to Radians/1
  angleOfAttack_deg/1 -> CYMDAAL_DA_ALFA/1, CYMDAL_DE_ALFA/1, CYMDAL_DE_ALFA1/1
  CYMDAL_DE_ALFA/1 -> Sum/1
  CYMDAL_DE_ALFA1/1 -> Sum/2
  Sum/1 -> Product/2
  Degrees to Radians/1 -> Product/1
  CYMDAAL_DA_ALFA/1 -> Product1/2
  Sign/1 -> Product1/1
  Product1/1 -> Sum1/1
  Product/1 -> Sum1/2
  Sum1/1 -> Product2/1
  eieff/1 -> Product2/2
  qacorr/1 -> CYMEDAI_QA_M/2
  mach_nd/1 -> CYMEDAI_QA_M/1
  CYMEDAI_QA_M/1 -> Product2/3

== system ADMIRE/Aircraft/Aerodynamics/YawMomentCoefficient/MachRegion1/Cymdaib/Cymdaib_ ==
  angleOfAttack_deg : Inport
  dAI : Inport  Port=2
  angleOfSideslip_deg : Inport  Port=3
  eieff : Inport  Port=4
  Abs : Abs
  Abs1 : Abs
  Abs2 : Abs
  CYMDABAL_ALFA : Lookup_n-D  NumberOfTableDimensions=1  BreakpointsForDimension1=admireDB.aerodata_asym_ext.CYMDABAL.breakpoints.ALFA  BreakpointsForDimension3=[5, 7]  Table=admireDB.aerodata_asym_ext.CYMDABAL.newTable  ExtrapMethod=Clip  InternalRulePriority=Speed  RndMeth=Simplest  InputSameDT=on
  Constant : Constant  Value=30
  Constant1 : Constant  Value=20
  Product : Product  Inputs=**/*/*
  Cymdaib : Outport
  wires:
  Product/1 -> Cymdaib/1
  angleOfAttack_deg/1 -> Abs/1
  CYMDABAL_ALFA/1 -> Product/1
  dAI/1 -> Abs1/1
  Abs/1 -> CYMDABAL_ALFA/1
  Abs1/1 -> Product/2
  Constant/1 -> Product/3
  angleOfSideslip_deg/1 -> Abs2/1
  Constant1/1 -> Product/5
  Abs2/1 -> Product/4
  eieff/1 -> Product/6

== system ADMIRE/Aircraft/Aerodynamics/YawMomentCoefficient/MachRegion1/Cymday/Cymday_ ==
  dAY : Inport
  angleOfAttack_deg : Inport  Port=2
  dEY : Inport  Port=3
  eoeff : Inport  Port=4
  qacorr : Inport  Port=5
  mach_nd : Inport  Port=6
  Abs : Abs
  CYMDAAL_DA_ALFA : Lookup_n-D  BreakpointsForDimension1=admireDB.aerodata_asym_ext.CYMDAAL.breakpoints.ALFA  BreakpointsForDimension2=admireDB.aerodata_asym_ext.CYMDAAL.breakpoints.DA  BreakpointsForDimension3=[5, 7]  Table=admireDB.aerodata_asym_ext.CYMDAAL.newTable  ExtrapMethod=Clip  InternalRulePriority=Speed  RndMeth=Simplest  InputSameDT=on
      settings: InputPortMap=u0,u1
  CYMDAL_DE_ALFA : Lookup_n-D  BreakpointsForDimension1=admireDB.aerodata_asym_ext.CYMDAL.breakpoints.ALFA  BreakpointsForDimension2=admireDB.aerodata_asym_ext.CYMDAL.breakpoints.DE  BreakpointsForDimension3=[5, 7]  Table=admireDB.aerodata_asym_ext.CYMDAL.newTable  ExtrapMethod=Clip  InternalRulePriority=Speed  RndMeth=Simplest  InputSameDT=on
      settings: InputPortMap=u0,u1
  CYMDAL_DE_ALFA1 : Lookup_n-D  BreakpointsForDimension1=admireDB.aerodata_asym_ext.CYMDAL.breakpoints.ALFA  BreakpointsForDimension2=admireDB.aerodata_asym_ext.CYMDAL.breakpoints.DE  BreakpointsForDimension3=[5, 7]  Table=admireDB.aerodata_asym_ext.CYMDAL.newTable  ExtrapMethod=Clip  InternalRulePriority=Speed  RndMeth=Simplest  InputSameDT=on
      settings: InputPortMap=u0,u1
  CYMEDAY_QA_M : Lookup_n-D  BreakpointsForDimension1=admireDB.aerodata_asym_ext.CYMEDAY.breakpoints.M  BreakpointsForDimension2=admireDB.aerodata_asym_ext.CYMEDAY.breakpoints.QA  BreakpointsForDimension3=[5, 7]  Table=admireDB.aerodata_asym_ext.CYMEDAY.newTable  ExtrapMethod=Clip  InternalRulePriority=Speed  RndMeth=Simplest  InputSameDT=on
      settings: InputPortMap=u0,u1
  Degrees to Radians : simulink_extras/Transformations/Degrees to Radians
  Product{,1..3} (4 alike) : Product
  Sign : Signum
  Sum : Sum  Inputs=|+-
  Sum1 : Sum  Inputs=|++
  Sum2 : Sum  Inputs=|++
  dE_cnst : Constant  Value=0.0
  Cymday : Outport
  wires:
  dEY/1 -> CYMDAL_DE_ALFA/2
  dE_cnst/1 -> CYMDAL_DE_ALFA1/2
  Product3/1 -> Sum2/2
  Sum2/1 -> Cymday/1
  CYMEDAY_QA_M/1 -> Product3/2
  mach_nd/1 -> CYMEDAY_QA_M/1
  qacorr/1 -> CYMEDAY_QA_M/2
  eoeff/1 -> Product2/2
  Sum1/1 -> Product2/1
  Product/1 -> Sum1/2
  Product1/1 -> Sum1/1
  Sign/1 -> Product1/1
  CYMDAAL_DA_ALFA/1 -> Product1/2
  Degrees to Radians/1 -> Product/1, Product3/1
  Sum/1 -> Product/2
  CYMDAL_DE_ALFA1/1 -> Sum/2
  CYMDAL_DE_ALFA/1 -> Sum/1
  angleOfAttack_deg/1 -> CYMDAAL_DA_ALFA/1, CYMDAL_DE_ALFA/1, CYMDAL_DE_ALFA1/1
  dAY/1 -> Abs/1, Sign/1, Degrees to Radians/1
  Abs/1 -> CYMDAAL_DA_ALFA/2
  Product2/1 -> Sum2/1

== system ADMIRE/Aircraft/Aerodynamics/YawMomentCoefficient/MachRegion1/Cymdayb/Cymdayb_ ==
  angleOfAttack_deg : Inport
  dAY : Inport  Port=2
  angleOfSideslip_deg : Inport  Port=3
  eoeff : Inport  Port=4
  Abs : Abs
  Abs1 : Abs
  Abs2 : Abs
  CYMDABAL_ALFA : Lookup_n-D  NumberOfTableDimensions=1  BreakpointsForDimension1=admireDB.aerodata_asym_ext.CYMDABAL.breakpoints.ALFA  BreakpointsForDimension3=[5, 7]  Table=admireDB.aerodata_asym_ext.CYMDABAL.newTable  ExtrapMethod=Clip  InternalRulePriority=Speed  RndMeth=Simplest  InputSameDT=on
  Constant : Constant  Value=30
  Constant1 : Constant  Value=20
  Product : Product  Inputs=**/*/*
  Cymdaib : Outport
  wires:
  eoeff/1 -> Product/6
  Abs2/1 -> Product/4
  Constant1/1 -> Product/5
  angleOfSideslip_deg/1 -> Abs2/1
  Constant/1 -> Product/3
  Abs1/1 -> Product/2
  Abs/1 -> CYMDABAL_ALFA/1
  dAY/1 -> Abs1/1
  CYMDABAL_ALFA/1 -> Product/1
  angleOfAttack_deg/1 -> Abs/1
  Product/1 -> Cymdaib/1

== system ADMIRE/Aircraft/Aerodynamics/YawMomentCoefficient/MachRegion1/Cymdna/Cymdna_ ==
  dNE : Inport
  angleOfAttack_deg : Inport  Port=2
  dNA : Inport  Port=3
  CYMDNAAL_DNE_ALFA : Lookup_n-D  BreakpointsForDimension1=admireDB.aerodata_asym_ext.CYMDNAAL.breakpoints.ALFA  BreakpointsForDimension2=admireDB.aerodata_asym_ext.CYMDNAAL.breakpoints.DNE  BreakpointsForDimension3=[5, 7]  Table=admireDB.aerodata_asym_ext.CYMDNAAL.newTable  ExtrapMethod=Clip  InternalRulePriority=Speed  RndMeth=Simplest  InputSameDT=on
      settings: InputPortMap=u0,u1
  Degrees to Radians : simulink_extras/Transformations/Degrees to Radians
  Product : Product  Inputs=**
  Cymdna : Outport
  wires:
  Product/1 -> Cymdna/1
  dNE/1 -> CYMDNAAL_DNE_ALFA/2
  angleOfAttack_deg/1 -> CYMDNAAL_DNE_ALFA/1
  dNA/1 -> Degrees to Radians/1
  CYMDNAAL_DNE_ALFA/1 -> Product/1
  Degrees to Radians/1 -> Product/2

== system ADMIRE/Aircraft/Aerodynamics/YawMomentCoefficient/MachRegion1/Cymdr/Cymdr_ ==
  angleOfAttack_deg : Inport
  dR : Inport  Port=2
  angleOfSideslip_deg : Inport  Port=3
  qacorr : Inport  Port=4
  mach_nd : Inport  Port=5
  CYMBDRAL_ALFA_DR_BETA : Lookup_n-D  NumberOfTableDimensions=3  BreakpointsForDimension1=admireDB.aerodata_asym_ext.CYMBDRAL.breakpoints.ALFA  BreakpointsForDimension2=admireDB.aerodata_asym_ext.CYMBDRAL.breakpoints.DR  BreakpointsForDimension3=admireDB.aerodata_asym_ext.CYMBDRAL.breakpoints.BETA  Table=admireDB.aerodata_asym_ext.CYMBDRAL.newTable  ExtrapMethod=Clip  InternalRulePriority=Speed  RndMeth=Simplest  InputSameDT=on
      settings: InputPortMap=u0,u1,u2
  CYMEDR_QA_M : Lookup_n-D  BreakpointsForDimension1=admireDB.aerodata_asym_ext.CYMEDR.breakpoints.M  BreakpointsForDimension2=admireDB.aerodata_asym_ext.CYMEDR.breakpoints.QA  BreakpointsForDimension3=[5, 7]  Table=admireDB.aerodata_asym_ext.CYMEDR.newTable  ExtrapMethod=Clip  InternalRulePriority=Speed  RndMeth=Simplest  InputSameDT=on
      settings: InputPortMap=u0,u1
  Product : Product
  Cymdr : Outport
  wires:
  angleOfSideslip_deg/1 -> CYMBDRAL_ALFA_DR_BETA/3
  Product/1 -> Cymdr/1
  qacorr/1 -> CYMEDR_QA_M/2
  mach_nd/1 -> CYMEDR_QA_M/1
  dR/1 -> CYMBDRAL_ALFA_DR_BETA/2
  angleOfAttack_deg/1 -> CYMBDRAL_ALFA_DR_BETA/1
  CYMEDR_QA_M/1 -> Product/2
  CYMBDRAL_ALFA_DR_BETA/1 -> Product/1

== system ADMIRE/Aircraft/Aerodynamics/YawMomentCoefficient/MachRegion1/Cymp/Cymp_ ==
  dN : Inport
  angleOfAttack_deg : Inport  Port=2
  qacorr : Inport  Port=3
  mach_nd : Inport  Port=4
  pc : Inport  Port=5
  CYMEP_QA_M : Lookup_n-D  BreakpointsForDimension1=admireDB.aerodata_asym_ext.CYMEP.breakpoints.M  BreakpointsForDimension2=admireDB.aerodata_asym_ext.CYMEP.breakpoints.QA  BreakpointsForDimension3=[5, 7]  Table=admireDB.aerodata_asym_ext.CYMEP.newTable  ExtrapMethod=Clip  InternalRulePriority=Speed  RndMeth=Simplest  InputSameDT=on
      settings: InputPortMap=u0,u1
  CYMPAL_DN_ALFA : Lookup_n-D  BreakpointsForDimension1=admireDB.aerodata_asym_ext.CYMPAL.breakpoints.ALFA  BreakpointsForDimension2=admireDB.aerodata_asym_ext.CYMPAL.breakpoints.DN  BreakpointsForDimension3=[5, 7]  Table=admireDB.aerodata_asym_ext.CYMPAL.newTable  ExtrapMethod=Clip  InternalRulePriority=Speed  RndMeth=Simplest  InputSameDT=on
      settings: InputPortMap=u0,u1
  Product : Product
  Sum : Sum  Inputs=|++
  Cymp : Outport
  wires:
  Sum/1 -> Product/1
  qacorr/1 -> CYMEP_QA_M/2
  mach_nd/1 -> CYMEP_QA_M/1
  dN/1 -> CYMPAL_DN_ALFA/2
  angleOfAttack_deg/1 -> CYMPAL_DN_ALFA/1
  CYMPAL_DN_ALFA/1 -> Sum/1
  CYMEP_QA_M/1 -> Sum/2
  pc/1 -> Product/2
  Product/1 -> Cymp/1

== system ADMIRE/Aircraft/Aerodynamics/YawMomentCoefficient/MachRegion1/Cympbeta/Cympbeta_ ==
  angleOfSideslip_deg : Inport
  angleOfAttack_deg : Inport  Port=2
  pc : Inport  Port=3
  Abs : Abs
  CYMPBA_BETA_ALFA : Lookup_n-D  BreakpointsForDimension1=admireDB.aerodata_asym_ext.CYMPBA.breakpoints.ALFA  BreakpointsForDimension2=admireDB.aerodata_asym_ext.CYMPBA.breakpoints.BETA  BreakpointsForDimension3=[5, 7]  Table=admireDB.aerodata_asym_ext.CYMPBA.newTable  ExtrapMethod=Clip  InternalRulePriority=Speed  RndMeth=Simplest  InputSameDT=on
      settings: InputPortMap=u0,u1
  Product : Product  Inputs=**
  Cympbeta : Outport
  wires:
  Product/1 -> Cympbeta/1
  pc/1 -> Product/2
  angleOfSideslip_deg/1 -> CYMPBA_BETA_ALFA/2
  angleOfAttack_deg/1 -> Abs/1
  CYMPBA_BETA_ALFA/1 -> Product/1
  Abs/1 -> CYMPBA_BETA_ALFA/1

== system ADMIRE/Aircraft/Aerodynamics/YawMomentCoefficient/MachRegion1/Cymr/Cymr_ ==
  dN : Inport
  angleOfAttack_deg : Inport  Port=2
  rc : Inport  Port=3
  mach_nd : Inport  Port=4
  qacorr : Inport  Port=5
  CYMER_M_QA : Lookup_n-D  BreakpointsForDimension1=admireDB.aerodata_asym_ext.CYMER.breakpoints.QA  BreakpointsForDimension2=admireDB.aerodata_asym_ext.CYMER.breakpoints.M  BreakpointsForDimension3=[5, 7]  Table=admireDB.aerodata_asym_ext.CYMER.newTable  ExtrapMethod=Clip  InternalRulePriority=Speed  RndMeth=Simplest  InputSameDT=on
      settings: InputPortMap=u0,u1
  CYMRAL_DN_ALFA : Lookup_n-D  BreakpointsForDimension1=admireDB.aerodata_asym_ext.CYMRAL.breakpoints.ALFA  BreakpointsForDimension2=admireDB.aerodata_asym_ext.CYMRAL.breakpoints.DN  BreakpointsForDimension3=[5, 7]  Table=admireDB.aerodata_asym_ext.CYMRAL.newTable  ExtrapMethod=Clip  InternalRulePriority=Speed  RndMeth=Simplest  InputSameDT=on
      settings: InputPortMap=u0,u1
  Product : Product  Inputs=***
  Cymr : Outport
  wires:
  CYMER_M_QA/1 -> Product/3
  mach_nd/1 -> CYMER_M_QA/2
  qacorr/1 -> CYMER_M_QA/1
  rc/1 -> Product/2
  Product/1 -> Cymr/1
  dN/1 -> CYMRAL_DN_ALFA/2
  angleOfAttack_deg/1 -> CYMRAL_DN_ALFA/1
  CYMRAL_DN_ALFA/1 -> Product/1

== system ADMIRE/Aircraft/Aerodynamics/YawMomentCoefficient/MachRegion1/Cymrbeta/Cymrbeta_ ==
  angleOfSideslip_deg : Inport
  angleOfAttack_deg : Inport  Port=2
  rc : Inport  Port=3
  Abs : Abs
  CYMRBA_BETA_ALFA : Lookup_n-D  BreakpointsForDimension1=admireDB.aerodata_asym_ext.CYMRBA.breakpoints.ALFA  BreakpointsForDimension2=admireDB.aerodata_asym_ext.CYMRBA.breakpoints.BETA  BreakpointsForDimension3=[5, 7]  Table=admireDB.aerodata_asym_ext.CYMRBA.newTable  ExtrapMethod=Clip  InternalRulePriority=Speed  RndMeth=Simplest  InputSameDT=on
      settings: InputPortMap=u0,u1
  Product : Product  Inputs=**
  Cymrbeta : Outport
  wires:
  CYMRBA_BETA_ALFA/1 -> Product/1
  Product/1 -> Cymrbeta/1
  rc/1 -> Product/2
  angleOfSideslip_deg/1 -> CYMRBA_BETA_ALFA/2
  angleOfAttack_deg/1 -> Abs/1
  Abs/1 -> CYMRBA_BETA_ALFA/1

== system ADMIRE/Aircraft/Aerodynamics/YawMomentCoefficient/MachRegion2/Cymbasic/Cymbasic_ ==
  angleOfAttack_deg : Inport
  tflow : Inport  Port=2
  Abs : Abs
  CYMZERO_ALFA : Lookup_n-D  NumberOfTableDimensions=1  BreakpointsForDimension1=admireDB.aerodata_asym_ext.CYMZERO.breakpoints.ALFA  BreakpointsForDimension3=[5, 7]  Table=admireDB.aerodata_asym_ext.CYMZERO.newTable  ExtrapMethod=Clip  InternalRulePriority=Speed  RndMeth=Simplest  InputSameDT=on
  Product : Product
  Cymbasic : Outport
  wires:
  Abs/1 -> CYMZERO_ALFA/1
  angleOfAttack_deg/1 -> Abs/1
  CYMZERO_ALFA/1 -> Product/1
  Product/1 -> Cymbasic/1
  tflow/1 -> Product/2

== system ADMIRE/Aircraft/Aerodynamics/YawMomentCoefficient/MachRegion2/Cymbcai/Cymbcai_ ==
  CAI : Inport
  angleOfAttack_deg : Inport  Port=2
  angleOfSideslip_deg : Inport  Port=3
  CYMBCAI_CAI_ALFA : Lookup_n-D  BreakpointsForDimension1=admireDB.aerodata_asym_ext.CYMBCAI.breakpoints.ALFA  BreakpointsForDimension2=admireDB.aerodata_asym_ext.CYMBCAI.breakpoints.CAI  BreakpointsForDimension3=[5, 7]  Table=admireDB.aerodata_asym_ext.CYMBCAI.newTable  ExtrapMethod=Clip  InternalRulePriority=Speed  RndMeth=Simplest  InputSameDT=on
      settings: InputPortMap=u0,u1
  Degrees to Radians : simulink_extras/Transformations/Degrees to Radians
  Product : Product  Inputs=**
  Cymbcai : Outport
  wires:
  Product/1 -> Cymbcai/1
  Degrees to Radians/1 -> Product/2
  angleOfSideslip_deg/1 -> Degrees to Radians/1
  CYMBCAI_CAI_ALFA/1 -> Product/1
  CAI/1 -> CYMBCAI_CAI_ALFA/2
  angleOfAttack_deg/1 -> CYMBCAI_CAI_ALFA/1

== system ADMIRE/Aircraft/Aerodynamics/YawMomentCoefficient/MachRegion2/Cymbde/Cymbde_ ==
  angleOfAttack_deg : Inport
  dEI : Inport  Port=2
  angleOfSideslip_deg : Inport  Port=3
  dEY : Inport  Port=4
  eieff : Inport  Port=5
  eoeff : Inport  Port=6
  Abs : Abs
  CYMDEB_ALFA_DE_BETA : Lookup_n-D  NumberOfTableDimensions=3  BreakpointsForDimension1=admireDB.aerodata_asym_ext.CYMDEB.breakpoints.ALFA  BreakpointsForDimension2=admireDB.aerodata_asym_ext.CYMDEB.breakpoints.DE  BreakpointsForDimension3=admireDB.aerodata_asym_ext.CYMDEB.breakpoints.BETA  Table=admireDB.aerodata_asym_ext.CYMDEB.newTable  ExtrapMethod=Clip  InternalRulePriority=Speed  RndMeth=Simplest  InputSameDT=on
      settings: InputPortMap=u0,u1,u2
  CYMDEB_ALFA_DE_BETA1 : Lookup_n-D  NumberOfTableDimensions=3  BreakpointsForDimension1=admireDB.aerodata_asym_ext.CYMDEB.breakpoints.ALFA  BreakpointsForDimension2=admireDB.aerodata_asym_ext.CYMDEB.breakpoints.DE  BreakpointsForDimension3=admireDB.aerodata_asym_ext.CYMDEB.breakpoints.BETA  Table=admireDB.aerodata_asym_ext.CYMDEB.newTable  ExtrapMethod=Clip  InternalRulePriority=Speed  RndMeth=Simplest  InputSameDT=on
      settings: InputPortMap=u0,u1,u2
  Product : Product  Inputs=**
  Product1 : Product  Inputs=**
  Product2 : Product
  Sign : Signum
  Sum : Sum  Inputs=|++
  Cymbde : Outport
  wires:
  Sign/1 -> Product2/1
  Product2/1 -> Cymbde/1
  Product1/1 -> Sum/2
  Product/1 -> Sum/1
  Sum/1 -> Product2/2
  eoeff/1 -> Product1/1
  eieff/1 -> Product/2
  CYMDEB_ALFA_DE_BETA1/1 -> Product1/2
  CYMDEB_ALFA_DE_BETA/1 -> Product/1
  Abs/1 -> CYMDEB_ALFA_DE_BETA1/3, CYMDEB_ALFA_DE_BETA/3
  angleOfSideslip_deg/1 -> Abs/1, Sign/1
  dEI/1 -> CYMDEB_ALFA_DE_BETA/2
  angleOfAttack_deg/1 -> CYMDEB_ALFA_DE_BETA1/1, CYMDEB_ALFA_DE_BETA/1
  dEY/1 -> CYMDEB_ALFA_DE_BETA1/2
